simulink model "Sim1"  (R2023a)
settings: Solver=VariableStepAuto  StartTime=0.0  StopTime=10.0  RelTol=1e-3
undefined symbols (not defined in the file or in its folder): A, B, K, Kr
settings Model: Creator=vince  LastModifiedBy=vince

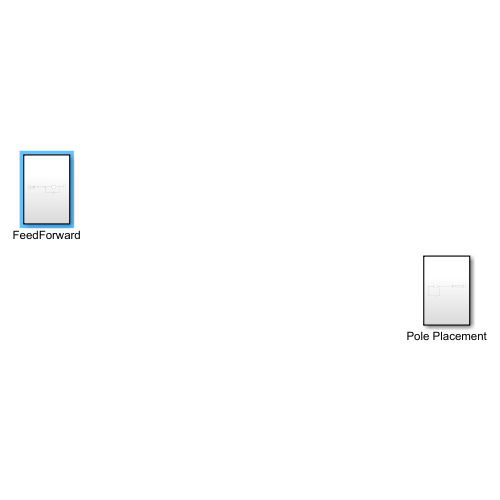
[thumbnail: Simulink's stored preview of the top-level diagram]
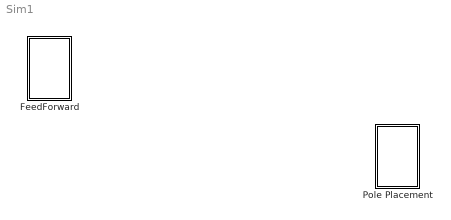
== system Sim1 ==
  FeedForward : Subsystem
  Pole Placement : Subsystem

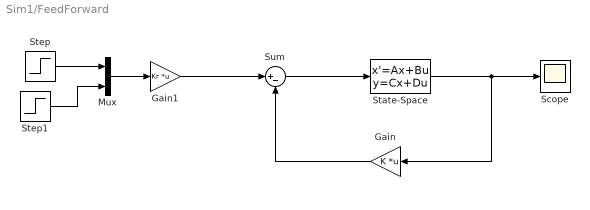
== system Sim1/FeedForward ==
  Gain : Gain  Gain=K  Multiplication=Matrix(K*u)
  Gain1 : Gain  Gain=Kr  Multiplication=Matrix(K*u)
  Mux : Mux  Inputs=2
  Scope : Scope
  State-Space : StateSpace  InitialCondition=0
  Step : Step  Time=0  SampleTime=0
  Step1 : Step  Time=0  SampleTime=0
  Sum : Sum  Inputs=|+-
  wires:
  Gain1/1 -> Sum/1
  Gain/1 -> Sum/2
  Sum/1 -> State-Space/1
  Step/1 -> Mux/1
  State-Space/1 -> Gain/1, Scope/1
  Step1/1 -> Mux/2
  Mux/1 -> Gain1/1

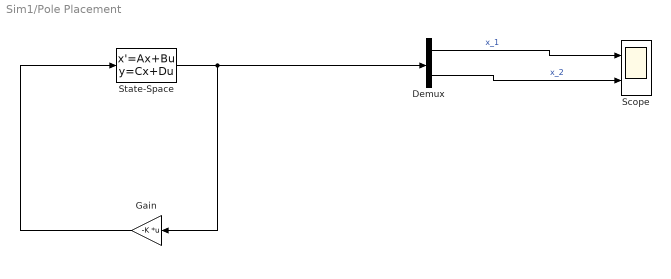
== system Sim1/Pole Placement ==
  Demux : Demux  Outputs=2
  Gain : Gain  Gain=-K  Multiplication=Matrix(K*u)
  Scope : Scope  NumInputPorts=2
  State-Space : StateSpace  A=A  B=B  C=eye(2)  D=[0;0]  InitialCondition=[1;-1;]
  wires:
  Gain/1 -> State-Space/1
  State-Space/1 -> Gain/1, Demux/1
  Demux/1 -> Scope/1  "x_1"
  Demux/2 -> Scope/2  "x_2"
